simulink model "Model_3DoF_Complete"  (R2024a)
settings: Solver=VariableStepAuto  StartTime=0.0  StopTime=6  RelTol=1e-3
model workspace: external: MATLAB File C:\Users\C27Derek.Weissinger\OneDrive - USAFA (AFAcademy.AF.edu)\Documents\Classes\Summer 26\Astro 499\Derek-Weissinger-GNC-Methods-2026\MATLAB + Simulink\vehicle_params.m (data not in the file)
values from neighbouring files (symbols this model uses):
  I = 0.048    [vehicle_params.m]
  Kd = 0.3    [vehicle_params.m]
  Ki = 0.01    [vehicle_params.m]
  Kp = 2    [vehicle_params.m]
  Lg = 0.28    [vehicle_params.m]
  m = 0.543    [vehicle_params.m]
  thetai = 5    [vehicle_params.m]
  Ts = 0.01    [vehicle_params.m]
libraries: simulink_extras x2, sharedtransform x1, eeGeneralControl x1
settings Model: Creator=C28Derek.Weissinger  LastModifiedBy=C28Derek.Weissinger

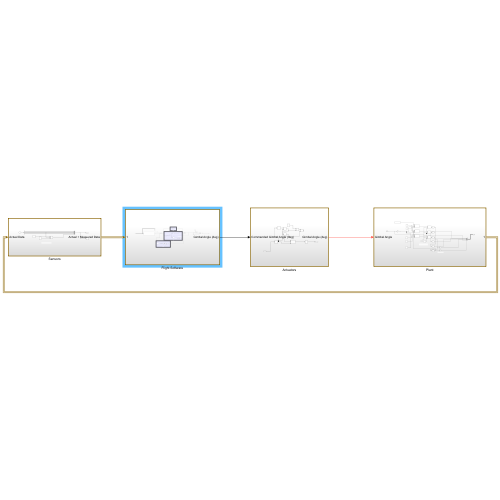
[thumbnail: Simulink's stored preview of the top-level diagram]
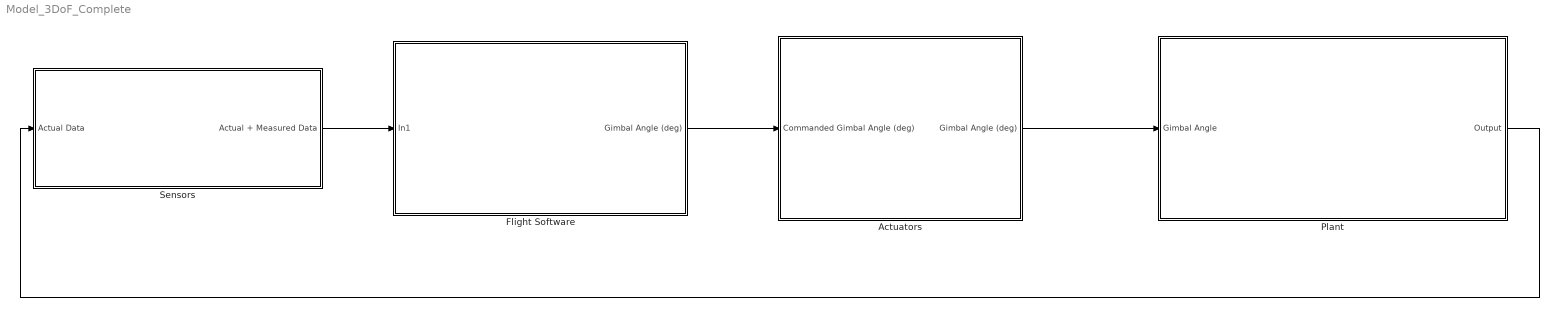
== system Model_3DoF_Complete ==
  Actuators : Subsystem
  Flight Software : Subsystem
  Plant : Subsystem
  Sensors : Subsystem
  wires:
  Plant/1(Output) -> Sensors/1(Actual Data)
  Sensors/1(Actual + Measured Data) -> Flight Software/1(In1)
  Flight Software/1(Gimbal Angle (deg)) -> Actuators/1(Commanded Gimbal Angle (deg))
  Actuators/1(Gimbal Angle (deg)) -> Plant/1(Gimbal Angle)

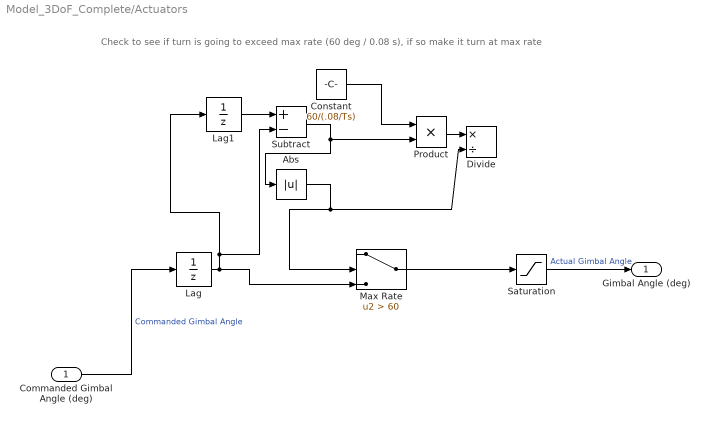
== system Model_3DoF_Complete/Actuators ==
  note: Check to see if turn is going to exceed max rate (60 deg / 0.08 s), if so make it turn at max rate
  Commanded Gimbal Angle (deg) : Inport
  Abs : Abs  SaturateOnIntegerOverflow=off
  Constant : Constant  Value=60/(.08/Ts)
  Divide : Product  Inputs=*/
  Lag : UnitDelay  SampleTime=Ts  HasFrameUpgradeWarning=on
  Lag1 : UnitDelay  SampleTime=0.08  HasFrameUpgradeWarning=on
  Max Rate : Switch  Criteria=u2 > Threshold  Threshold=60  SaturateOnIntegerOverflow=off  InputSameDT=off
  Product : Product
  Saturation : Saturate  UpperLimit=5  LowerLimit=-5
  Subtract : Sum  Inputs=+-
  Gimbal Angle (deg) : Outport
  wires:
  Commanded Gimbal Angle (deg)/1 -> Lag/1  "Commanded Gimbal Angle"
  Saturation/1 -> Gimbal Angle (deg)/1  "Actual Gimbal Angle"
  Lag/1 -> Max Rate/3, Subtract/2, Lag1/1
  Lag1/1 -> Subtract/1
  Subtract/1 -> Abs/1, Product/2
  Abs/1 -> Max Rate/2, Divide/2
  Constant/1 -> Product/1
  Product/1 -> Divide/1
  Max Rate/1 -> Saturation/1

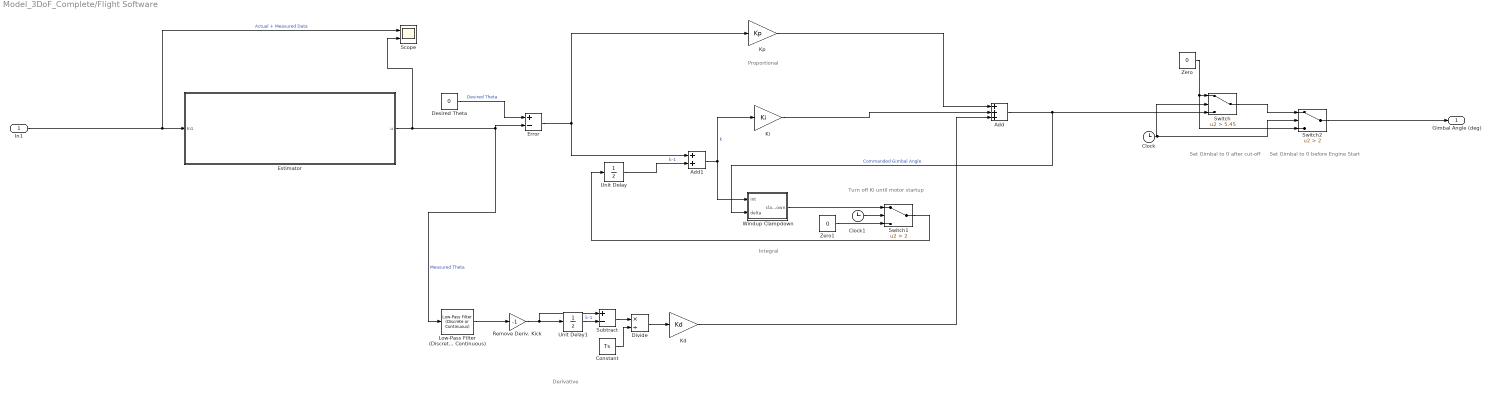
== system Model_3DoF_Complete/Flight Software ==
  note: Turn off Ki until motor startup
  note: Integral
  note: Proportional
  note: Derivative
  note: Set Gimbal to 0 before Engine Start
  note: Set Gimbal to 0 after cut-off
  In1 : Inport
  Add : Sum  Inputs=+++
  Add1 : Sum
  Clock : Clock
  Clock1 : Clock
  Constant : Constant  Value=Ts
  Desired Theta : Constant  Value=0
  Divide : Product  Inputs=*/
  Error : Sum  Inputs=+-
  Estimator : Subsystem
  Kd : Gain  Gain=Kd
  Ki : Gain  Gain=Ki
  Kp : Gain  Gain=Kp
  Low-Pass Filter (Discrete or Continuous) : eeGeneralControl/Low-Pass Filter (Discrete or Continuous)  K=1  T=2*Ts  B=inf  A=-inf  init_option=Inherited from block input  x0=0  Ts=-1
  Remove Deriv. Kick : Gain  Gain=-1
  Scope : Scope  NumInputPorts=2
  Subtract : Sum  Inputs=+-
  Switch : Switch  Criteria=u2 > Threshold  Threshold=5.45  SaturateOnIntegerOverflow=off  InputSameDT=off
  Switch1 : Switch  Criteria=u2 > Threshold  Threshold=2  SaturateOnIntegerOverflow=off  InputSameDT=off
  Switch2 : Switch  Criteria=u2 > Threshold  Threshold=2  SaturateOnIntegerOverflow=off  InputSameDT=off
  Unit Delay : UnitDelay  SampleTime=Ts  HasFrameUpgradeWarning=on
  Unit Delay1 : UnitDelay  SampleTime=Ts  HasFrameUpgradeWarning=on
  Windup Clampdown : MATLAB Function  TreatAsAtomicUnit=on
  Zero : Constant  Value=0  OutDataTypeStr=Inherit: Inherit via back propagation
  Zero1 : Constant  Value=0  OutDataTypeStr=Inherit: Inherit via back propagation
  Gimbal Angle (deg) : Outport
  wires:
  In1/1 -> Scope/1, Estimator/1(In1)  "Actual + Measured Data"
  Kp/1 -> Add/1
  Kd/1 -> Add/3
  Desired Theta/1 -> Error/1  "Desired Theta"
  Add/1 -> Windup Clampdown/2(delta), Switch/3  "Commanded Gimbal Angle"
  Unit Delay/1 -> Add1/2  "k-1"
  Add1/1 -> Windup Clampdown/1(Int), Ki/1  "k"
  Subtract/1 -> Divide/1
  Constant/1 -> Divide/2
  Divide/1 -> Kd/1
  Unit Delay1/1 -> Subtract/2  "k-1"
  Error/1 -> Add1/1, Kp/1
  Estimator/1(u) -> Scope/2, Low-Pass Filter (Discrete or Continuous)/1, Error/2  "Measured Theta"
  Clock/1 -> Switch2/2, Switch/2
  Zero/1 -> Switch2/3, Switch/1
  Switch/1 -> Switch2/1
  Windup Clampdown/1(clampdown) -> Switch1/1
  Switch2/1 -> Gimbal Angle (deg)/1
  Ki/1 -> Add/2
  Switch1/1 -> Unit Delay/1
  Zero1/1 -> Switch1/3
  Clock1/1 -> Switch1/2
  Low-Pass Filter (Discrete or Continuous)/1 -> Remove Deriv. Kick/1
  Remove Deriv. Kick/1 -> Subtract/1, Unit Delay1/1

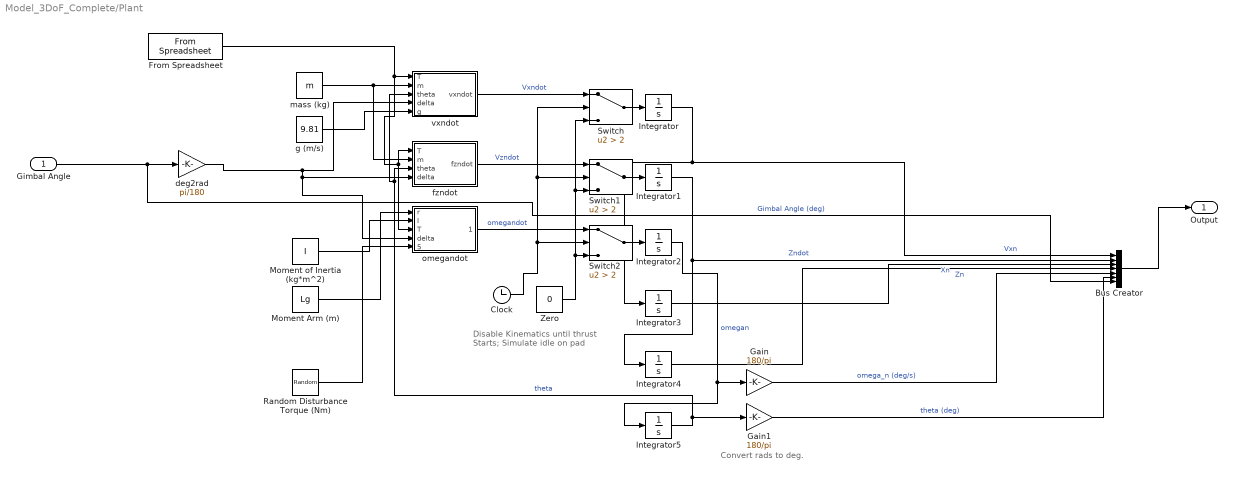
== system Model_3DoF_Complete/Plant ==
  note: Disable Kinematics until thrust
      | Starts; Simulate idle on pad
  note: Convert rads to deg.
  Gimbal Angle : Inport
  Bus Creator : BusCreator  Inputs=7
  Clock : Clock
  From Spreadsheet : FromSpreadsheet  FileName=Estes_F15.csv  SheetName=Estes_F15  ExtrapolationAfterLastDataPoint=Ground value
  Gain : Gain  Gain=180/pi
  Gain1 : Gain  Gain=180/pi
  Integrator{,1..4} (5 alike) : Integrator
  Integrator5 : Integrator  InitialCondition=deg2rad(thetai)
  Moment Arm (m) : Constant  Value=Lg
  Moment of Inertia (kg*m^2) : Constant  Value=I
  Random Disturbance Torque (Nm) : RandomNumber  Variance=.02  Seed=1  SampleTime=0.1
  Switch : Switch  Criteria=u2 > Threshold  Threshold=2  SaturateOnIntegerOverflow=off  InputSameDT=off
  Switch1 : Switch  Criteria=u2 > Threshold  Threshold=2  SaturateOnIntegerOverflow=off  InputSameDT=off
  Switch2 : Switch  Criteria=u2 > Threshold  Threshold=2  SaturateOnIntegerOverflow=off  InputSameDT=off
  Zero : Constant  Value=0  OutDataTypeStr=Inherit: Inherit via back propagation
  deg2rad : Gain  Gain=pi/180
  fzndot : MATLAB Function  TreatAsAtomicUnit=on
  g (m/s) : Constant  Value=9.81
  mass (kg) : Constant  Value=m
  omegandot : MATLAB Function  TreatAsAtomicUnit=on
  vxndot : MATLAB Function  TreatAsAtomicUnit=on
  Output : Outport
  wires:
  Integrator/1 -> Integrator3/1, Bus Creator/1  "Vxn"
  vxndot/1(vxndot) -> Switch/1  "Vxndot"
  fzndot/1(fzndot) -> Switch1/1  "Vzndot"
  Integrator2/1 -> Integrator5/1, Gain/1  "omegan"
  omegandot/1(omegandot) -> Switch2/1  "omegandot"
  Integrator3/1 -> Bus Creator/3  "Xn"
  Integrator1/1 -> Integrator4/1, Bus Creator/2  "Zndot"
  Integrator4/1 -> Bus Creator/4  "Zn"
  From Spreadsheet/1 -> omegandot/3(T), fzndot/1(T), vxndot/1(T)
  mass (kg)/1 -> fzndot/2(m), vxndot/2(m)
  g (m/s)/1 -> vxndot/5(g)
  Integrator5/1 -> Gain1/1, fzndot/3(theta), vxndot/3(theta)  "theta"
  Moment Arm (m)/1 -> omegandot/1(r)
  Moment of Inertia (kg*m^2)/1 -> omegandot/2(I)
  Bus Creator/1 -> Output/1
  deg2rad/1 -> omegandot/4(delta), fzndot/4(delta), vxndot/4(delta)
  Gimbal Angle/1 -> Bus Creator/7, deg2rad/1  "Gimbal Angle (deg)"
  Gain/1 -> Bus Creator/5  "omega_n (deg/s)"
  Gain1/1 -> Bus Creator/6  "theta (deg)"
  Random Disturbance Torque (Nm)/1 -> omegandot/5(envtorque)
  Switch/1 -> Integrator/1
  Switch2/1 -> Integrator2/1
  Switch1/1 -> Integrator1/1
  Clock/1 -> Switch/2, Switch1/2, Switch2/2
  Zero/1 -> Switch/3, Switch1/3, Switch2/3

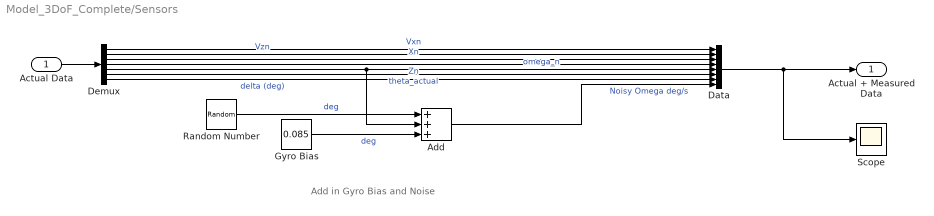
== system Model_3DoF_Complete/Sensors ==
  note: Add in Gyro Bias and Noise
  Actual Data : Inport
  Add : Sum  Inputs=+++
  Data : BusCreator  Inputs=8
  Demux : Demux  Outputs=7
  Gyro Bias : Constant  Value=0.085
  Random Number : RandomNumber  Variance=.25  SampleTime=0.01
  Scope : Scope
  Actual + Measured Data : Outport
  wires:
  Actual Data/1 -> Demux/1
  Demux/5 -> Add/2, Data/5  "omega_n"
  Random Number/1 -> Add/1  "deg"
  Gyro Bias/1 -> Add/3  "deg"
  Add/1 -> Data/8  "Noisy Omega deg/s"
  Demux/1 -> Data/1  "Vxn"
  Demux/2 -> Data/2  "Vzn"
  Demux/3 -> Data/3  "Xn"
  Demux/4 -> Data/4  "Zn"
  Demux/6 -> Data/6  "theta_actual"
  Data/1 -> Scope/1, Actual + Measured Data/1
  Demux/7 -> Data/7  "delta (deg)"

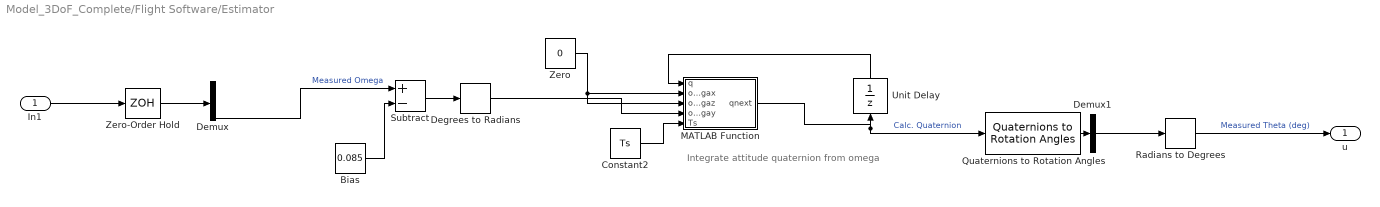
== system Model_3DoF_Complete/Flight Software/Estimator ==
  note: Integrate attitude quaternion from omega
  In1 : Inport
  Bias : Constant  Value=0.085  SampleTime=-1
  Constant2 : Constant  Value=Ts
  Degrees to Radians : simulink_extras/Transformations/Degrees to Radians
  Demux : Demux  Outputs=8
  Demux1 : Demux  Outputs=3
  MATLAB Function : MATLAB Function  TreatAsAtomicUnit=on
  Quaternions to Rotation Angles : sharedtransform/Quaternions to Rotation Angles  rotationOrder=ZYX  aMode=aMode
  Radians to Degrees : simulink_extras/Transformations/Radians to Degrees
  Subtract : Sum  Inputs=+-
  Unit Delay : UnitDelay  InitialCondition=eul2quat([0,deg2rad(thetai),0])  SampleTime=Ts  HasFrameUpgradeWarning=on
  Zero : Constant  Value=0  OutDataTypeStr=Inherit: Inherit via back propagation
  Zero-Order Hold : ZeroOrderHold  SampleTime=Ts
  u : Outport
  wires:
  In1/1 -> Zero-Order Hold/1
  Quaternions to Rotation Angles/1 -> Demux1/1
  Demux1/2 -> Radians to Degrees/1
  Radians to Degrees/1 -> u/1  "Measured Theta (deg)"
  Unit Delay/1 -> MATLAB Function/1(q)
  Demux/8 -> Subtract/1  "Measured Omega"
  Zero/1 -> MATLAB Function/3(omegaz), MATLAB Function/2(omegax)
  MATLAB Function/1(qnext) -> Quaternions to Rotation Angles/1, Unit Delay/1  "Calc. Quaternion"
  Subtract/1 -> Degrees to Radians/1
  Bias/1 -> Subtract/2
  Constant2/1 -> MATLAB Function/5(Ts)
  Degrees to Radians/1 -> MATLAB Function/4(omegay)
  Zero-Order Hold/1 -> Demux/1

== matlab function Model_3DoF_Complete/Plant/fzndot ==
  data: T input; fzndot output; m input; theta input; delta input
function fzndot = fcn(T, m, theta, delta)
   fzndot = (T/m) * (sin(theta - delta));
end

== matlab function Model_3DoF_Complete/Plant/vxndot ==
  data: T input; vxndot output; m input; theta input; delta input; g input
function vxndot = fcn(T, m, theta, delta, g)
   vxndot = (T/m) * (cos(theta - delta)) - g;
end

== matlab function Model_3DoF_Complete/Plant/omegandot ==
  data: r input; omegandot output; I input; T input; delta input; envtorque input
function omegandot = fcn(r, I, T, delta, envtorque)

omegandot = (r/I) * T * delta + (envtorque/I);

end

== matlab function Model_3DoF_Complete/Flight Software/Windup Clampdown ==
  data: Int input; clampdown output; delta input
function clampdown = fcn(Int,delta)
if abs(Int) > 5 && Int*delta >0
        clampdown = 0;
else
    clampdown = Int;
end
end

== matlab function Model_3DoF_Complete/Flight Software/Estimator/MATLAB Function ==
  data: q input; omegax input; omegaz input; omegay input; qnext output; Ts input
function qnext = fcn(q, omegax, omegaz, omegay, Ts)
%Closed form of quaternion integrator, as found on 
% https://ahrs.readthedocs.io/en/latest/filters/angular.html

omegamatrix = [0 -omegax -omegay -omegaz;
               omegax 0 omegaz -omegay;
               omegay -omegaz 0 omegax;
               omegaz omegay -omegax 0];

% qmatrix = [q0 -q3 q2 q1;
%           q3 q0 -q1 q2;
%           -q2 q1 q0 q3;
%           -q1 -q2 -q3 q0];
% omega = [omegax; omegay; omegaz; 0];
% qdot = 0.5 * matrix * omega;

qdot = 0.5 * omegamatrix * q;
qnext = q + qdot*Ts;
qnext = qnext/norm(qnext);

end
